simulink model "sampleModel1793"  (R2023a)
settings: Solver=VariableStepAuto  StartTime=0.0  StopTime=10.0  RelTol=1e-3
libraries: hdlsllib x5, simulink x1
settings Model: Creator=user1  LastModifiedBy=user1

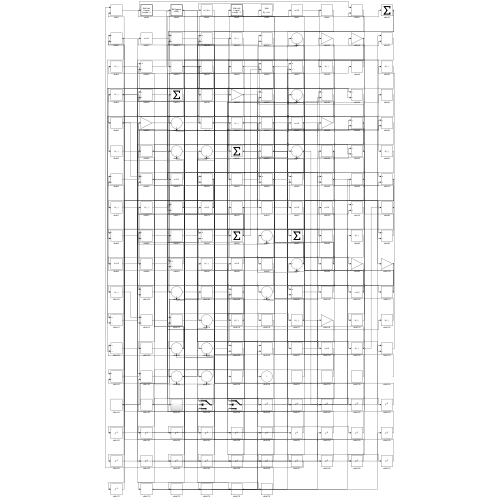
[thumbnail: Simulink's stored preview of the top-level diagram]
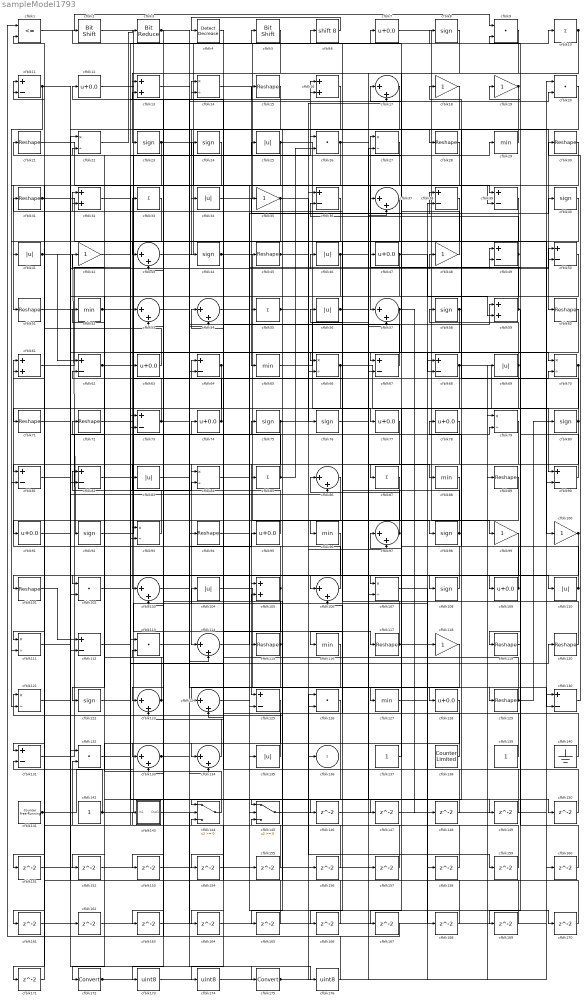
== system sampleModel1793 ==
  cfblk1 : RelationalOperator  Operator=<=  OutDataTypeStr=boolean  InputSameDT=off
  cfblk{10,33,55,85,87} (5 alike) : Sum  Inputs=+
  cfblk{18..19,35,42,48,99..100,118} (8 alike) : Gain
  cfblk{15,21,28,30..31,45,51,60,71..72,89,94,101,115,117,119..120,129} (18 alike) : Reshape
  cfblk{9,20,26,102,113,126,132} (7 alike) : DotProduct  OutDataTypeStr=Inherit: Inherit via internal rule
  cfblk{17,37,43,53..54,57,86,97,103,106,114,123..124,133..134} (15 alike) : Sum  Inputs=|++
  cfblk{25,34,41,46,56,69,83,104,110,135} (10 alike) : Abs  SaturateOnIntegerOverflow=off
  cfblk{13,16,32,59,61,105} (6 alike) : Sum
  cfblk{14,22,27,66,70,79,84,93,107,111,121} (11 alike) : Product  Inputs=*/  RndMeth=Zero  SaturateOnIntegerOverflow=on
  cfblk{8,23..24,40,44,58,75..76,80,92,98,108,122} (13 alike) : Signum
  cfblk{7,12,47,63,74,77..78,91,95,109,128} (11 alike) : Bias  Bias=0.0  SaturateOnIntegerOverflow=off
  cfblk{11,36,38..39,49..50,62,64,67..68,73,81..82,90,112,125,130..131} (18 alike) : Sum  Inputs=+-
  cfblk{29,52,65,88,96,116,127} (7 alike) : MinMax
  cfblk137 : Constant  SampleTime=-1
  cfblk138 : hdlsllib/Sources/Counter Limited  uplimit=7  tsamp=-1
  cfblk139 : Constant  SampleTime=-1
  cfblk140 : Ground
  cfblk141 : hdlsllib/Sources/Counter Free-Running  NumBits=16  tsamp=-1
  cfblk142 : Constant  SampleTime=-1
  cfblk143 : Subsystem
      settings: LibrarySourceBlock=|
      | hdlsllib/Ports &
      | Subsystems/Subsystem
  cfblk144 : Switch  SaturateOnIntegerOverflow=off  InputSameDT=off
  cfblk145 : Switch  SaturateOnIntegerOverflow=off  InputSameDT=off
  cfblk{146..171} (26 alike) : Delay  SampleTime=1
  cfblk172 : DataTypeConversion  SaturateOnIntegerOverflow=off  RndMeth=Floor
  cfblk173 : DataTypeConversion  OutDataTypeStr=uint8  SaturateOnIntegerOverflow=off  RndMeth=Floor
  cfblk174 : DataTypeConversion  OutDataTypeStr=uint8  SaturateOnIntegerOverflow=off  RndMeth=Floor
  cfblk175 : DataTypeConversion  SaturateOnIntegerOverflow=off  RndMeth=Floor
  cfblk176 : DataTypeConversion  OutDataTypeStr=uint8  SaturateOnIntegerOverflow=off  RndMeth=Floor
  cfblk2 : hdlsllib/Logic and Bit Operations/Bit Shift  mode=Shift Left Logical  N=0
  cfblk3 : hdlsllib/Logic and Bit Operations/Bit Reduce  mode=AND
  cfblk4 : simulink/Logic and Bit Operations/Detect Decrease  vinit=0.0  OutDataTypeStr=boolean
      settings: LibrarySourceBlock=|
      | hdlsllib/Logic and Bit
      | Operations/Detect
      | Decrease
  cfblk5 : hdlsllib/Logic and Bit Operations/Bit Shift  mode=Shift Left Logical  N=0
  cfblk6 : ArithShift  BitShiftNumber=8
  cfblk136 : Outport  VectorParamsAs1DForOutWhenUnconnected=off
  wires:
  cfblk25/1 -> cfblk77/1, cfblk164/1
  cfblk47/1 -> cfblk59/2, cfblk173/1
  cfblk75/1 -> cfblk121/1, cfblk70/2, cfblk161/1
  cfblk92/1 -> cfblk46/1
  cfblk78/1 -> cfblk114/1
  cfblk57/1 -> cfblk73/2, cfblk148/1
  cfblk98/1 -> cfblk56/1, cfblk31/1
  cfblk6/1 -> cfblk4/1
  cfblk58/1 -> cfblk144/1, cfblk64/2
  cfblk2/1 -> cfblk117/1
  cfblk105/1 -> cfblk124/1, cfblk24/1
  cfblk106/1 -> cfblk61/1
  cfblk5/1 -> cfblk23/1
  cfblk1/1 -> cfblk9/1
  cfblk30/1 -> cfblk57/1
  cfblk33/1 -> cfblk101/1
  cfblk77/1 -> cfblk125/1
  cfblk131/1 -> cfblk74/1
  cfblk143/1(Out1) -> cfblk175/1
  cfblk52/1 -> cfblk16/1, cfblk25/1
  cfblk10/1 -> cfblk13/1, cfblk107/2
  cfblk65/1 -> cfblk29/1
  cfblk43/1 -> cfblk7/1
  cfblk9/1 -> cfblk67/1
  cfblk44/1 -> cfblk98/1, cfblk170/1
  cfblk95/1 -> cfblk33/1
  cfblk7/1 -> cfblk99/1
  cfblk101/1 -> cfblk112/1
  cfblk53/1 -> cfblk106/1
  cfblk129/1 -> cfblk32/1, cfblk80/1
  cfblk76/1 -> cfblk128/1
  cfblk82/1 -> cfblk103/1
  cfblk141/1 -> cfblk104/1, cfblk120/1
  cfblk22/1 -> cfblk3/1
  cfblk142/1 -> cfblk68/1, cfblk131/2, cfblk84/2
  cfblk74/1 -> cfblk71/1, cfblk52/1
  cfblk26/1 -> cfblk65/1, cfblk111/2, cfblk39/2
  cfblk50/1 -> cfblk116/1
  cfblk103/1 -> cfblk95/1
  cfblk16/1 -> cfblk55/1
  cfblk24/1 -> cfblk123/1
  cfblk15/1 -> cfblk44/1
  cfblk116/1 -> cfblk125/2
  cfblk59/1 -> cfblk27/1, cfblk119/1
  cfblk41/1 -> cfblk92/1, cfblk62/1
  cfblk14/1 -> cfblk45/1
  cfblk23/1 -> cfblk81/1, cfblk37/2, cfblk135/1
  cfblk68/1 -> cfblk90/1, cfblk91/1
  cfblk20/1 -> cfblk105/1
  cfblk104/1 -> cfblk136/1
  cfblk12/1 -> cfblk60/1
  cfblk89/1 -> cfblk115/1
  cfblk97/1 -> cfblk86/1, cfblk26/1
  cfblk28/1 -> cfblk112/2
  cfblk144/1 -> cfblk72/1
  cfblk130/1 -> cfblk30/1
  cfblk48/1 -> cfblk21/1
  cfblk46/1 -> cfblk102/1, cfblk149/1
  cfblk115/1 -> cfblk124/2, cfblk32/2
  cfblk145/1 -> cfblk69/1
  cfblk73/1 -> cfblk59/1, cfblk62/2
  cfblk86/1 -> cfblk93/1
  cfblk66/1 -> cfblk100/1, cfblk84/1
  cfblk90/1 -> cfblk19/1
  cfblk137/1 -> cfblk47/1
  cfblk69/1 -> cfblk58/1, cfblk103/2
  cfblk40/1 -> cfblk85/1
  cfblk111/1 -> cfblk50/1
  cfblk123/1 -> cfblk82/1, cfblk22/2
  cfblk91/1 -> cfblk75/1
  cfblk11/1 -> cfblk81/2, cfblk86/2
  cfblk34/1 -> cfblk8/1
  cfblk83/1 -> cfblk54/2
  cfblk85/1 -> cfblk53/1, cfblk43/2, cfblk26/2
  cfblk84/1 -> cfblk50/2
  cfblk100/1 -> cfblk107/1, cfblk169/1
  cfblk56/1 -> cfblk6/1, cfblk68/2, cfblk110/1, cfblk88/1
  cfblk93/1 -> cfblk42/1
  cfblk18/1 -> cfblk43/1
  cfblk54/1 -> cfblk40/1
  cfblk120/1 -> cfblk5/1
  cfblk140/1 -> cfblk97/1
  cfblk55/1 -> cfblk76/1, cfblk17/2
  cfblk45/1 -> cfblk97/2, cfblk70/1
  cfblk109/1 -> cfblk2/1, cfblk78/1
  cfblk135/1 -> cfblk14/1
  cfblk21/1 -> cfblk63/1
  cfblk139/1 -> cfblk14/2
  cfblk29/1 -> cfblk28/1
  cfblk36/1 -> cfblk133/1
  cfblk79/1 -> cfblk134/1
  cfblk108/1 -> cfblk35/1
  cfblk122/1 -> cfblk16/2
  cfblk113/1 -> cfblk20/2
  cfblk70/1 -> cfblk87/1, cfblk127/1
  cfblk119/1 -> cfblk49/1
  cfblk110/1 -> cfblk37/1, cfblk17/1
  cfblk117/1 -> cfblk64/1, cfblk150/1
  cfblk60/1 -> cfblk83/1
  cfblk51/1 -> cfblk10/1
  cfblk132/1 -> cfblk79/2
  cfblk81/1 -> cfblk132/1
  cfblk35/1 -> cfblk121/2, cfblk159/1
  cfblk39/1 -> cfblk96/1
  cfblk13/1 -> cfblk129/1
  cfblk112/1 -> cfblk93/2
  cfblk62/1 -> cfblk49/2, cfblk66/1
  cfblk99/1 -> cfblk145/1
  cfblk80/1 -> cfblk18/1, cfblk111/1
  cfblk114/1 -> cfblk38/1
  cfblk67/1 -> cfblk12/1
  cfblk31/1 -> cfblk90/2, cfblk66/2
  cfblk138/1 -> cfblk106/2
  cfblk133/1 -> cfblk94/1, cfblk15/1
  cfblk134/1 -> cfblk113/2
  cfblk126/1 -> cfblk172/1
  cfblk63/1 -> cfblk11/1
  cfblk61/1 -> cfblk48/1
  cfblk38/1 -> cfblk51/1
  cfblk19/1 -> cfblk82/2, cfblk108/1
  cfblk27/1 -> cfblk41/1
  cfblk64/1 -> cfblk122/1, cfblk151/1
  cfblk3/1 -> cfblk130/2, cfblk133/2, cfblk39/1
  cfblk127/1 -> cfblk118/1
  cfblk87/1 -> cfblk131/1
  cfblk102/1 -> cfblk109/1
  cfblk72/1 -> cfblk36/1
  cfblk32/1 -> cfblk34/1
  cfblk49/1 -> cfblk145/2, cfblk36/2, cfblk102/2
  cfblk124/1 -> cfblk146/1
  cfblk146/1 -> cfblk20/1
  cfblk42/1 -> cfblk147/1
  cfblk147/1 -> cfblk79/1
  cfblk148/1 -> cfblk54/1
  cfblk149/1 -> cfblk123/2
  cfblk150/1 -> cfblk113/1
  cfblk151/1 -> cfblk134/2
  cfblk128/1 -> cfblk152/1
  cfblk152/1 -> cfblk57/2
  cfblk17/1 -> cfblk153/1
  cfblk153/1 -> cfblk53/2
  cfblk8/1 -> cfblk154/1
  cfblk154/1 -> cfblk67/2
  cfblk94/1 -> cfblk155/1
  cfblk155/1 -> cfblk61/2
  cfblk156/1 -> cfblk105/2
  cfblk157/1 -> cfblk132/2
  cfblk158/1 -> cfblk73/1
  cfblk159/1 -> cfblk144/2
  cfblk160/1 -> cfblk9/2
  cfblk161/1 -> cfblk38/2
  cfblk71/1 -> cfblk162/1
  cfblk162/1 -> cfblk130/1
  cfblk125/1 -> cfblk163/1
  cfblk163/1 -> cfblk114/2
  cfblk164/1 -> cfblk27/2
  cfblk118/1 -> cfblk165/1
  cfblk165/1 -> cfblk22/1
  cfblk37/1 -> cfblk166/1
  cfblk166/1 -> cfblk144/3
  cfblk88/1 -> cfblk167/1
  cfblk167/1 -> cfblk1/1
  cfblk107/1 -> cfblk168/1
  cfblk168/1 -> cfblk13/2
  cfblk169/1 -> cfblk145/3
  cfblk170/1 -> cfblk1/2
  cfblk96/1 -> cfblk171/1
  cfblk171/1 -> cfblk11/2
  cfblk172/1 -> cfblk158/1, cfblk157/1, cfblk156/1
  cfblk173/1 -> cfblk126/1
  cfblk4/1 -> cfblk174/1
  cfblk174/1 -> cfblk126/2
  cfblk175/1 -> cfblk160/1, cfblk89/1
  cfblk121/1 -> cfblk176/1
  cfblk176/1 -> cfblk143/1(In1)

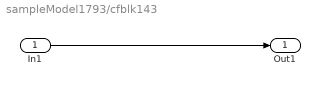
== system sampleModel1793/cfblk143 ==
  In1 : Inport
  Out1 : Outport
  wires:
  In1/1 -> Out1/1
